simulink model "sintonia_PID_exemplo"  (R2018a)
settings: Solver=ode45  StartTime=0.0  StopTime=7  RelTol=1e-3
settings Model: Creator=fernandopassold  LastModifiedBy=fernandopassold

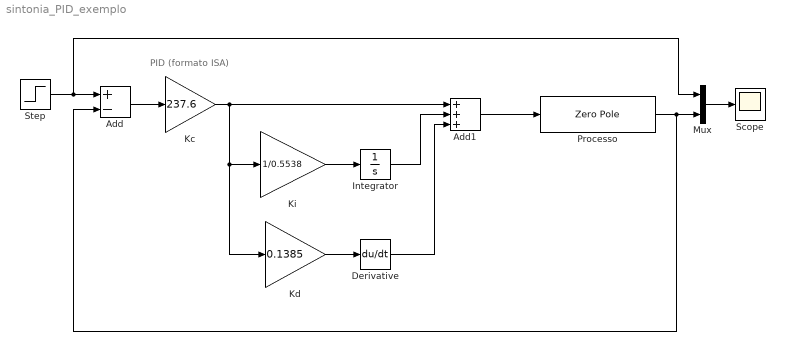
== system sintonia_PID_exemplo ==
  note: PID (formato ISA)
  Add : Sum  Inputs=+-
  Add1 : Sum  Inputs=+++
  Derivative : Derivative
  Integrator : Integrator
  Kc : Gain  Gain=237.6
  Kd : Gain  Gain=0.1385
  Ki : Gain  Gain=1/0.5538
  Mux : Mux  Inputs=2
  Processo : ZeroPole  Zeros=[ ]  Poles=[-1 -2 -10]
  Scope : Scope
  Step : Step  SampleTime=0
  wires:
  Add/1 -> Kc/1
  Kc/1 -> Kd/1, Ki/1, Add1/1
  Ki/1 -> Integrator/1
  Kd/1 -> Derivative/1
  Integrator/1 -> Add1/2
  Derivative/1 -> Add1/3
  Add1/1 -> Processo/1
  Processo/1 -> Add/2, Mux/2
  Step/1 -> Mux/1, Add/1
  Mux/1 -> Scope/1
